simulink model "hx_NTU_sim"  (R2017b)
settings: Solver=VariableStepAuto  StartTime=0.0  StopTime=0  RelTol=1e-3
undefined symbols (not defined in the file): P, rho, T
libraries: thermochemical x9
settings Model: Creator=fferrucc  LastModifiedBy=fferrucc

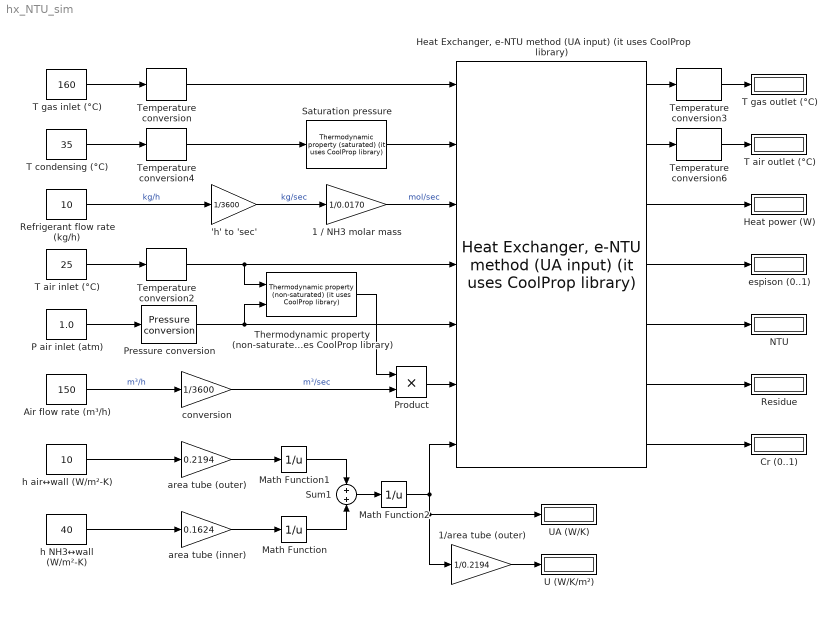
== system hx_NTU_sim ==
  'h' to 'sec' : Gain  Gain=1/3600
  1 / NH3 molar mass : Gain  Gain=1/0.0170
  1/area tube (outer) : Gain  Gain=1/0.2194
  Air flow rate (m³/h) : Constant  Value=150
  Cr (0..1) : Display
  "Heat Exchanger, e-NTU method (UA input) (it uses CoolProp library)" : thermochemical/Heat exchangers/Heat Exchanger, e-NTU method (UA input) (it uses CoolProp library)  fluidName_1=Ammonia  fluidName_2=Air  flowType=Cross-flow, both mixed
      settings: SourceProductName=@ Thermochemical
  "Heat power (W) " : Display
  Math Function : Math  Operator=reciprocal  SaturateOnIntegerOverflow=on
  Math Function1 : Math  Operator=reciprocal  SaturateOnIntegerOverflow=on
  Math Function2 : Math  Operator=reciprocal  SaturateOnIntegerOverflow=on
  NTU : Display
  "P air inlet (atm) " : Constant  Value=1.0
  Pressure conversion : thermochemical/Conversions/Pressure conversion  sel=atm --> bar
      settings: SourceProductName=@ Thermochemical
  Product : Product
  Refrigerant flow rate (kg/h) : Constant  Value=10
  Residue : Display
  Saturation pressure : thermochemical/Thermodynamic fluid properties/Thermodynamic  property (saturated) (it uses CoolProp library)  sel=P(T) (bar)  fluid=Ammonia  ref=NBP: h=0, s=0 for saturated liquid at 1 atmosphere  reciprocVar=-1
      settings: SourceProductName=@ Thermochemical
  Sum1 : Sum
  T air inlet (°C) : Constant  Value=25
  T air outlet (°C) : Display
  T condensing (°C) : Constant  Value=35
  T gas inlet (°C) : Constant  Value=160
  "T gas outlet (°C) " : Display
  Temperature conversion : thermochemical/Conversions/Temperature conversion  sel=°C --> K
      settings: SourceProductName=@ Thermochemical
  Temperature conversion2 : thermochemical/Conversions/Temperature conversion  sel=°C --> K
      settings: SourceProductName=@ Thermochemical
  Temperature conversion3 : thermochemical/Conversions/Temperature conversion  sel=K --> °C
      settings: SourceProductName=@ Thermochemical
  Temperature conversion4 : thermochemical/Conversions/Temperature conversion  sel=°C --> K
      settings: SourceProductName=@ Thermochemical
  Temperature conversion6 : thermochemical/Conversions/Temperature conversion  sel=K --> °C
      settings: SourceProductName=@ Thermochemical
  Thermodynamic property (non-saturated) (it uses CoolProp library) : thermochemical/Thermodynamic fluid properties/Thermodynamic  property (non-saturated) (it uses CoolProp library)  sel=rho(T,P)  fluid=Air  ref=NBP: h=0, s=0 for saturated liquid at 1 atmosphere  reciprocVar=-1
      settings: SourceProductName=@ Thermochemical
  U (W/K/m²) : Display
  UA (W/K) : Display
  area tube (inner) : Gain  Gain=0.1624
  area tube (outer) : Gain  Gain=0.2194
  conversion : Gain  Gain=1/3600
  espison (0..1) : Display
  h NH3↔wall (W/m²-K) : Constant  Value=40
  h air↔wall (W/m²-K) : Constant  Value=10
  wires:
  T gas inlet (°C)/1 -> Temperature conversion/1
  Temperature conversion3/1 -> "T gas outlet (°C) "/1
  1/area tube (outer)/1 -> U (W/K/m²)/1
  Temperature conversion/1 -> "Heat Exchanger, e-NTU method (UA input) (it uses CoolProp library)"/1
  T condensing (°C)/1 -> Temperature conversion4/1
  Temperature conversion4/1 -> Saturation pressure/1
  Saturation pressure/1 -> "Heat Exchanger, e-NTU method (UA input) (it uses CoolProp library)"/2
  Refrigerant flow rate (kg/h)/1 -> 'h' to 'sec'/1  "kg/h"
  T air inlet (°C)/1 -> Temperature conversion2/1
  "P air inlet (atm) "/1 -> Pressure conversion/1
  "Heat Exchanger, e-NTU method (UA input) (it uses CoolProp library)"/3 -> "Heat power (W) "/1
  "Heat Exchanger, e-NTU method (UA input) (it uses CoolProp library)"/5 -> NTU/1
  "Heat Exchanger, e-NTU method (UA input) (it uses CoolProp library)"/4 -> espison (0..1)/1
  "Heat Exchanger, e-NTU method (UA input) (it uses CoolProp library)"/1 -> Temperature conversion3/1
  "Heat Exchanger, e-NTU method (UA input) (it uses CoolProp library)"/2 -> Temperature conversion6/1
  Temperature conversion6/1 -> T air outlet (°C)/1
  "Heat Exchanger, e-NTU method (UA input) (it uses CoolProp library)"/6 -> Residue/1
  "Heat Exchanger, e-NTU method (UA input) (it uses CoolProp library)"/7 -> Cr (0..1)/1
  1 / NH3 molar mass/1 -> "Heat Exchanger, e-NTU method (UA input) (it uses CoolProp library)"/3  "mol/sec"
  'h' to 'sec'/1 -> 1 / NH3 molar mass/1  "kg/sec"
  Temperature conversion2/1 -> "Heat Exchanger, e-NTU method (UA input) (it uses CoolProp library)"/4, Thermodynamic property (non-saturated) (it uses CoolProp library)/1
  Pressure conversion/1 -> "Heat Exchanger, e-NTU method (UA input) (it uses CoolProp library)"/5, Thermodynamic property (non-saturated) (it uses CoolProp library)/2
  h NH3↔wall (W/m²-K)/1 -> area tube (inner)/1
  h air↔wall (W/m²-K)/1 -> area tube (outer)/1
  area tube (inner)/1 -> Math Function/1
  area tube (outer)/1 -> Math Function1/1
  Sum1/1 -> Math Function2/1
  Math Function2/1 -> 1/area tube (outer)/1, UA (W/K)/1, "Heat Exchanger, e-NTU method (UA input) (it uses CoolProp library)"/7
  Air flow rate (m³/h)/1 -> conversion/1  "m³/h"
  conversion/1 -> Product/2  "m³/sec"
  Product/1 -> "Heat Exchanger, e-NTU method (UA input) (it uses CoolProp library)"/6
  Thermodynamic property (non-saturated) (it uses CoolProp library)/1 -> Product/1
  Math Function1/1 -> Sum1/1
  Math Function/1 -> Sum1/2
